simulink subsystem "voc"  (R2022a)
settings: Solver=VariableStepAuto  StartTime=0.0  StopTime=10.0  RelTol=1e-3
undefined symbols (not defined in the file): ALPHA, BETA, OCV_1, OCV_2, OCV_3, OCV_4, OCV_5, OCV_6, OCV_ALPHA, OCV_BETA, OCV_GAMMA, OCV_V0, OCV_VL, T_REF
settings Model: Creator=Cristobal  LastModifiedBy=Cristobal

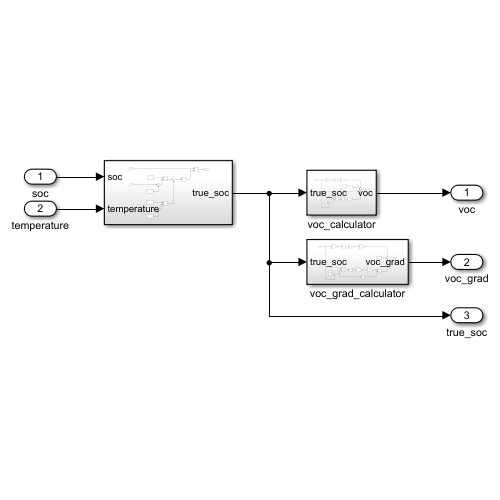
[thumbnail: Simulink's stored preview of the top-level diagram]
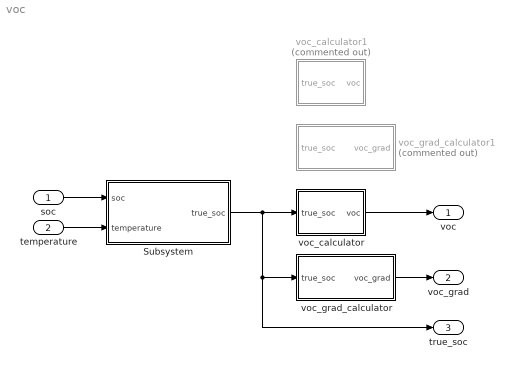
== system voc ==
  soc : Inport
  temperature : Inport  Port=2
  Subsystem : Subsystem
  voc_calculator : Subsystem
  voc_calculator1 : Subsystem  Commented=on
  voc_grad_calculator : Subsystem
  voc_grad_calculator1 : Subsystem  Commented=on
  voc : Outport
  voc_grad : Outport  Port=2
  true_soc : Outport  Port=3
  wires:
  voc_grad_calculator/1(voc_grad) -> voc_grad/1
  voc_calculator/1(voc) -> voc/1
  Subsystem/1(true_soc) -> voc_calculator/1(true_soc), voc_grad_calculator/1(true_soc), true_soc/1
  temperature/1 -> Subsystem/2(temperature)
  soc/1 -> Subsystem/1(soc)

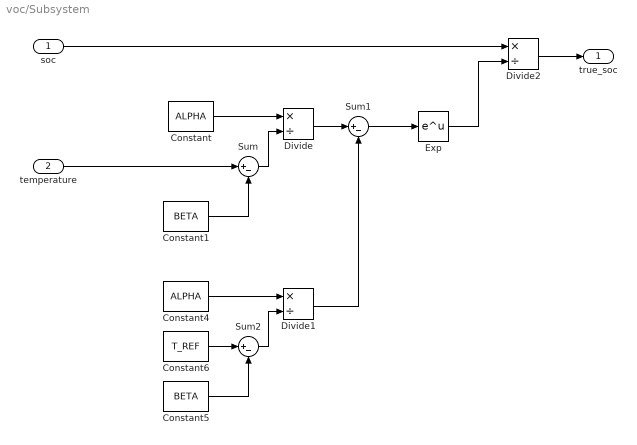
== system voc/Subsystem ==
  soc : Inport
  temperature : Inport  Port=2
  Constant : Constant  Value=ALPHA
  Constant1 : Constant  Value=BETA
  Constant4 : Constant  Value=ALPHA
  Constant5 : Constant  Value=BETA
  Constant6 : Constant  Value=T_REF
  Divide : Product  Inputs=*/
  Divide1 : Product  Inputs=*/
  Divide2 : Product  Inputs=*/
  Exp : Math
  Sum : Sum  Inputs=|+-
  Sum1 : Sum  Inputs=|+-
  Sum2 : Sum  Inputs=|+-
  true_soc : Outport
  wires:
  Divide2/1 -> true_soc/1
  soc/1 -> Divide2/1
  Constant5/1 -> Sum2/2
  Sum2/1 -> Divide1/2
  Sum/1 -> Divide/2
  Divide/1 -> Sum1/1
  Constant1/1 -> Sum/2
  Constant4/1 -> Divide1/1
  temperature/1 -> Sum/1
  Sum1/1 -> Exp/1
  Exp/1 -> Divide2/2
  Divide1/1 -> Sum1/2
  Constant/1 -> Divide/1
  Constant6/1 -> Sum2/1

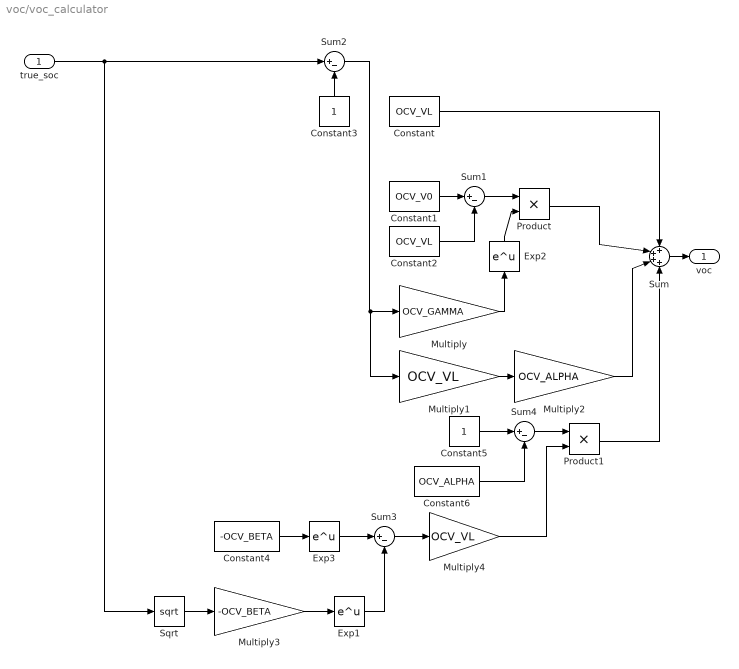
== system voc/voc_calculator ==
  true_soc : Inport
  Constant : Constant  Value=OCV_VL
  Constant1 : Constant  Value=OCV_V0
  Constant2 : Constant  Value=OCV_VL
  Constant3 : Constant
  Constant4 : Constant  Value=-OCV_BETA
  Constant5 : Constant
  Constant6 : Constant  Value=OCV_ALPHA
  Exp1 : Math
  Exp2 : Math
  Exp3 : Math
  Multiply : Gain  Gain=OCV_GAMMA
  Multiply1 : Gain  Gain=OCV_VL
  Multiply2 : Gain  Gain=OCV_ALPHA
  Multiply3 : Gain  Gain=-OCV_BETA
  Multiply4 : Gain  Gain=OCV_VL
  Product : Product
  Product1 : Product
  Sqrt : Sqrt
  Sum : Sum  Inputs=++++
  Sum{1..4} (4 alike) : Sum  Inputs=|+-
  voc : Outport
  wires:
  Sum/1 -> voc/1
  Product1/1 -> Sum/4
  Multiply4/1 -> Product1/2
  Sum4/1 -> Product1/1
  Constant6/1 -> Sum4/2
  Constant5/1 -> Sum4/1
  Sum3/1 -> Multiply4/1
  Exp3/1 -> Sum3/1
  Constant4/1 -> Exp3/1
  Exp1/1 -> Sum3/2
  Multiply3/1 -> Exp1/1
  Sqrt/1 -> Multiply3/1
  Multiply2/1 -> Sum/3
  Multiply1/1 -> Multiply2/1
  Product/1 -> Sum/2
  Exp2/1 -> Product/2
  Multiply/1 -> Exp2/1
  Sum2/1 -> Multiply/1, Multiply1/1
  Constant3/1 -> Sum2/2
  true_soc/1 -> Sum2/1, Sqrt/1
  Sum1/1 -> Product/1
  Constant2/1 -> Sum1/2
  Constant1/1 -> Sum1/1
  Constant/1 -> Sum/1

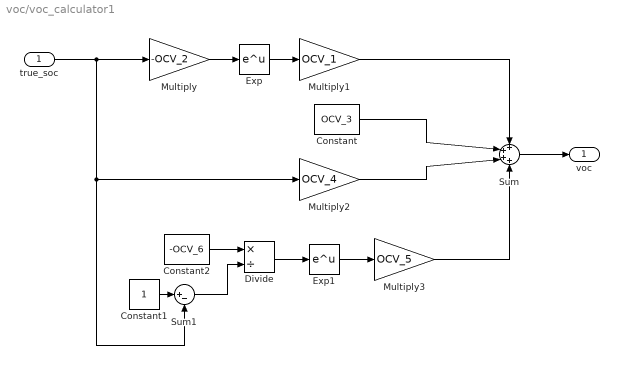
== system voc/voc_calculator1 ==
  true_soc : Inport
  Constant : Constant  Value=OCV_3
  Constant1 : Constant
  Constant2 : Constant  Value=-OCV_6
  Divide : Product  Inputs=*/
  Exp : Math
  Exp1 : Math
  Multiply : Gain  Gain=-OCV_2
  Multiply1 : Gain  Gain=OCV_1
  Multiply2 : Gain  Gain=OCV_4
  Multiply3 : Gain  Gain=OCV_5
  Sum : Sum  Inputs=++++
  Sum1 : Sum  Inputs=|+-
  voc : Outport
  wires:
  true_soc/1 -> Sum1/2, Multiply2/1, Multiply/1
  Multiply/1 -> Exp/1
  Exp/1 -> Multiply1/1
  Constant1/1 -> Sum1/1
  Sum1/1 -> Divide/2
  Constant2/1 -> Divide/1
  Divide/1 -> Exp1/1
  Multiply1/1 -> Sum/1
  Constant/1 -> Sum/2
  Multiply2/1 -> Sum/3
  Multiply3/1 -> Sum/4
  Sum/1 -> voc/1
  Exp1/1 -> Multiply3/1

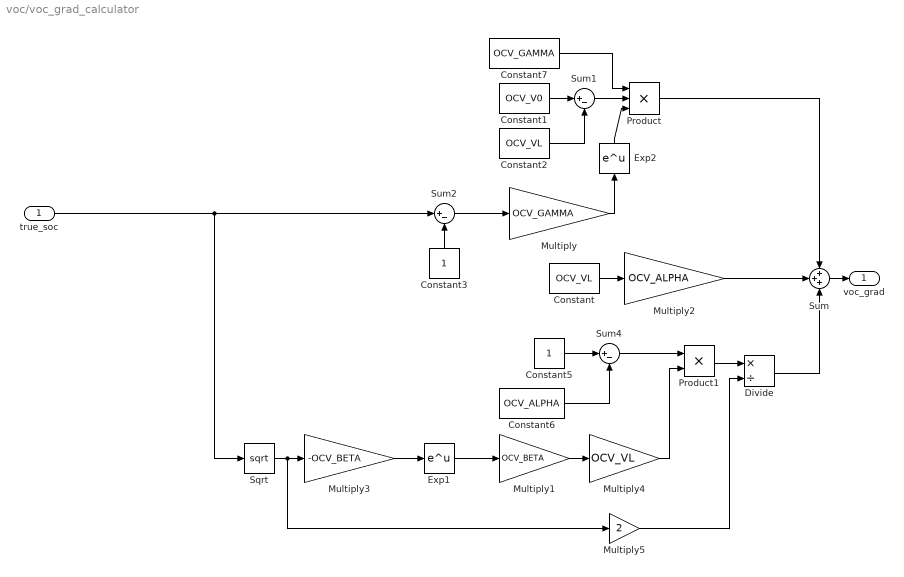
== system voc/voc_grad_calculator ==
  true_soc : Inport
  Constant : Constant  Value=OCV_VL
  Constant1 : Constant  Value=OCV_V0
  Constant2 : Constant  Value=OCV_VL
  Constant3 : Constant
  Constant5 : Constant
  Constant6 : Constant  Value=OCV_ALPHA
  Constant7 : Constant  Value=OCV_GAMMA
  Divide : Product  Inputs=*/
  Exp1 : Math
  Exp2 : Math
  Multiply : Gain  Gain=OCV_GAMMA
  Multiply1 : Gain  Gain=OCV_BETA
  Multiply2 : Gain  Gain=OCV_ALPHA
  Multiply3 : Gain  Gain=-OCV_BETA
  Multiply4 : Gain  Gain=OCV_VL
  Multiply5 : Gain  Gain=2
  Product : Product  Inputs=3
  Product1 : Product
  Sqrt : Sqrt
  Sum : Sum  Inputs=+++
  Sum1 : Sum  Inputs=|+-
  Sum2 : Sum  Inputs=|+-
  Sum4 : Sum  Inputs=|+-
  voc_grad : Outport
  wires:
  Divide/1 -> Sum/3
  Multiply5/1 -> Divide/2
  Product1/1 -> Divide/1
  Multiply1/1 -> Multiply4/1
  Multiply2/1 -> Sum/2
  Constant7/1 -> Product/1
  Product/1 -> Sum/1
  Sum1/1 -> Product/2
  Exp2/1 -> Product/3
  Multiply/1 -> Exp2/1
  Constant6/1 -> Sum4/2
  Multiply3/1 -> Exp1/1
  Sum/1 -> voc_grad/1
  Sum2/1 -> Multiply/1
  Constant3/1 -> Sum2/2
  Constant2/1 -> Sum1/2
  Constant5/1 -> Sum4/1
  Constant1/1 -> Sum1/1
  Sqrt/1 -> Multiply3/1, Multiply5/1
  Constant/1 -> Multiply2/1
  Multiply4/1 -> Product1/2
  Sum4/1 -> Product1/1
  true_soc/1 -> Sum2/1, Sqrt/1
  Exp1/1 -> Multiply1/1

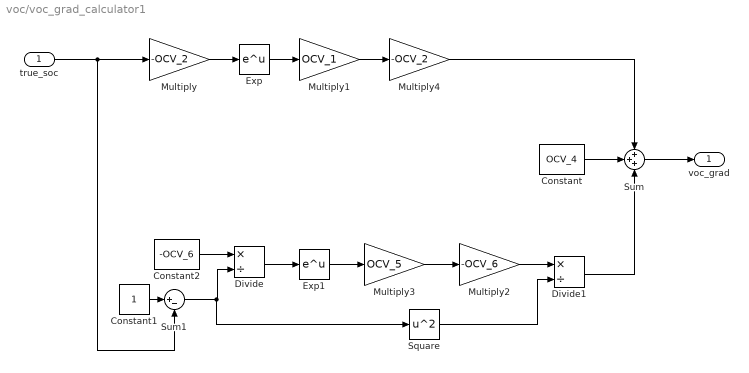
== system voc/voc_grad_calculator1 ==
  true_soc : Inport
  Constant : Constant  Value=OCV_4
  Constant1 : Constant
  Constant2 : Constant  Value=-OCV_6
  Divide : Product  Inputs=*/
  Divide1 : Product  Inputs=*/
  Exp : Math
  Exp1 : Math
  Multiply : Gain  Gain=-OCV_2
  Multiply1 : Gain  Gain=OCV_1
  Multiply2 : Gain  Gain=-OCV_6
  Multiply3 : Gain  Gain=OCV_5
  Multiply4 : Gain  Gain=-OCV_2
  Square : Math  Operator=square
  Sum : Sum  Inputs=+++
  Sum1 : Sum  Inputs=|+-
  voc_grad : Outport
  wires:
  Multiply/1 -> Exp/1
  Exp/1 -> Multiply1/1
  Multiply1/1 -> Multiply4/1
  Constant/1 -> Sum/2
  Sum/1 -> voc_grad/1
  Multiply4/1 -> Sum/1
  Constant2/1 -> Divide/1
  Divide/1 -> Exp1/1
  true_soc/1 -> Sum1/2, Multiply/1
  Sum1/1 -> Square/1, Divide/2
  Exp1/1 -> Multiply3/1
  Constant1/1 -> Sum1/1
  Multiply3/1 -> Multiply2/1
  Multiply2/1 -> Divide1/1
  Square/1 -> Divide1/2
  Divide1/1 -> Sum/3
